simulink model "ENV_hardcoded"  (R2024b)
settings: Solver=FixedStepDiscrete  StartTime=0.0  StopTime=10.0  FixedStep=0.001  RelTol=1e-3
libraries: stm32blockslib x54, canmsglib x29, simulink x7, stm32f4xxblockslib x1
(part 3 of 5)

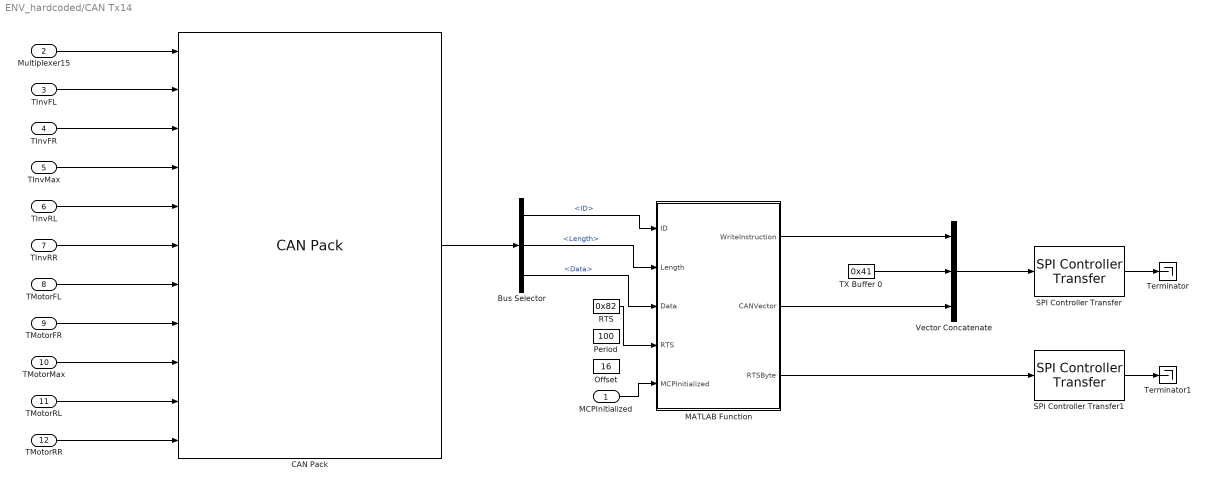
== system ENV_hardcoded/CAN Tx14 ==
  MCPInitialized : Inport  SampleTime=.001
  Multiplexer15 : Inport  Port=2
  TInvFL : Inport  Port=3
  TInvFR : Inport  Port=4
  TInvMax : Inport  Port=5
  TInvRL : Inport  Port=6
  TInvRR : Inport  Port=7
  TMotorFL : Inport  Port=8
  TMotorFR : Inport  Port=9
  TMotorMax : Inport  Port=10
  TMotorRL : Inport  Port=11
  TMotorRR : Inport  Port=12
  Bus Selector : BusSelector  OutputSignals=ID,Length,Data
  CAN Pack : canmsglib/CAN Pack  CANdbFile=C:\Users\William\Downloads\VCUSTM32\BaselineControls\CAN\CAN3_baseline.dbc  MsgList=Etas_Signals_15  MsgName=Etas_Signals_15  MsgIDType=Standard (11-bit identifier)  MsgIdentifier=2017  CANIDInput=off  MsgLength=8  Remote=off  ApplyMinMax=off  BusOutput=on  SignalInfo={'Multiplexer15','62','2','LE','unsigned','Multiplexor','0','1','0','0','3';'TInvFL','10','10','LE','unsigned','Multiplexed','1','0.1','0','0','102.3';'TInvFR','20','10','LE','unsigned','Multiplexed','1','0.1','0','0','102.3';'TInvMax','30','10','LE','unsigned','Multiplexed','1','0.1','0','0','102.3';'TInvRL','40','10','LE','unsigned','Multiplexed','1','0.1','0','0','102.3';'TInvRR','0','10','LE','unsigned','Multiplexed','1','0.1','0','0','102.3';'TMotorFL','12','11','LE','unsigned','Multiplexed','0','0.1','0','0','204.7';'TMotorFR','0','11','LE','unsigned','Multiplexed','0','0.1','0','0','204.7';'TMotorMax','45','11','LE','unsigned','Multiplexed','0','0.1','0','0','204.7';'TMotorRL','23','11','LE','unsigned','Multiplexed','0','0.1','0','0','204.7';'TMotorRR','34','11','LE','unsigned','Multiplexed','0','0.1','0','0','204.7'}
      settings: LibrarySourceBlock=stmutilitieslib/CAN Pack  DataFormat=CANdb specified signals
  MATLAB Function : MATLAB Function  TreatAsAtomicUnit=on
  Offset : Constant  Value=16  OutDataTypeStr=uint16  SampleTime=.001
  Period : Constant  Value=100  OutDataTypeStr=uint16  SampleTime=.001
  RTS : Constant  Value=0x82  OutDataTypeStr=uint8  SampleTime=.001
  SPI Controller Transfer : stm32blockslib/SPI Controller Transfer  Priority=1  SPIModuleSelect=SPI1  ClockPolarity=Low  ClockPhase=1 Edge  SPIModule=uint32(0)  Mode=Master  BusSpeed=uint32(1000000)  FirstBitToTransfer=Most significant bit (MSB)  ClockMode=0  BlockFunction=Transfer  EnableRegisterAddress=off  RegisterAddress=0  OutputDataType=uint8  OutputDataLength=1  OutputStatus=off  BlockingMode=off  Timeout=0.01  DataBits=8  UseCustomSSPin=Explicit GPIO calls  ActiveLowSSPin=Active low  Port_Select=GPIOA  Pin=4
      settings: LibrarySourceBlock=stm32h7xxblockslib/SPI Controller Transfer
  SPI Controller Transfer1 : stm32blockslib/SPI Controller Transfer  Priority=2  SPIModuleSelect=SPI1  ClockPolarity=Low  ClockPhase=1 Edge  SPIModule=uint32(0)  Mode=Master  BusSpeed=uint32(1000000)  FirstBitToTransfer=Most significant bit (MSB)  ClockMode=0  BlockFunction=Transfer  EnableRegisterAddress=off  RegisterAddress=0  OutputDataType=uint8  OutputDataLength=1  OutputStatus=off  BlockingMode=off  Timeout=0.01  DataBits=8  UseCustomSSPin=Explicit GPIO calls  ActiveLowSSPin=Active low  Port_Select=GPIOA  Pin=4
      settings: LibrarySourceBlock=stm32h7xxblockslib/SPI Controller Transfer
  TX Buffer 0 : Constant  Value=0x41  OutDataTypeStr=uint8  SampleTime=.001
  Terminator : Terminator
  Terminator1 : Terminator
  Vector Concatenate : Concatenate  NumInputs=3
  wires:
  TInvFL/1 -> CAN Pack/2
  Multiplexer15/1 -> CAN Pack/1
  TInvFR/1 -> CAN Pack/3
  TInvMax/1 -> CAN Pack/4
  TInvRL/1 -> CAN Pack/5
  TInvRR/1 -> CAN Pack/6
  TMotorFL/1 -> CAN Pack/7
  TMotorFR/1 -> CAN Pack/8
  TMotorMax/1 -> CAN Pack/9
  TMotorRL/1 -> CAN Pack/10
  TMotorRR/1 -> CAN Pack/11
  CAN Pack/1 -> Bus Selector/1
  SPI Controller Transfer/1 -> Terminator/1
  Bus Selector/1 -> MATLAB Function/1(ID)  "<ID>"
  Bus Selector/3 -> MATLAB Function/3(Data)  "<Data>"
  Vector Concatenate/1 -> SPI Controller Transfer/1
  Bus Selector/2 -> MATLAB Function/2(Length)  "<Length>"
  SPI Controller Transfer1/1 -> Terminator1/1
  MATLAB Function/2(CANVector) -> Vector Concatenate/3
  TX Buffer 0/1 -> Vector Concatenate/2
  MATLAB Function/3(RTSByte) -> SPI Controller Transfer1/1
  RTS/1 -> MATLAB Function/4(RTS)
  MCPInitialized/1 -> MATLAB Function/5(MCPInitialized)
  MATLAB Function/1(WriteInstruction) -> Vector Concatenate/1

== system ENV_hardcoded/CAN Tx15 ==
  MCPInitialized : Inport  SampleTime=.001
  NInvDTCFL : Inport  Port=2
  NInvDTCFR : Inport  Port=3
  NInvDTCRL : Inport  Port=4
  NInvDTCRR : Inport  Port=5
  TCellMax : Inport  Port=6
  VCellDelta : Inport  Port=7
  Bus Selector : BusSelector  OutputSignals=ID,Length,Data
  CAN Pack : canmsglib/CAN Pack  CANdbFile=C:\Users\William\Downloads\VCUSTM32\BaselineControls\CAN\CAN3_baseline.dbc  MsgList=Etas_Signals_16  MsgName=Etas_Signals_16  MsgIDType=Standard (11-bit identifier)  MsgIdentifier=2018  CANIDInput=off  MsgLength=8  Remote=off  ApplyMinMax=off  BusOutput=on  SignalInfo={'NInvDTCFL','12','12','LE','unsigned','Standard','0','1','0','0','4095';'NInvDTCFR','24','12','LE','unsigned','Standard','0','1','0','0','4095';'NinvDTCRL','36','12','LE','unsigned','Standard','0','1','0','0','4095';'NinvDTCRR','0','12','LE','unsigned','Standard','0','1','0','0','4095';'TCellMax','48','10','LE','unsigned','Standard','0','0.1','0','0','102.3';'VCellDelta','58','6','LE','unsigned','Standard','0','0.01','0','0','0.63'}
      settings: LibrarySourceBlock=stmutilitieslib/CAN Pack  DataFormat=CANdb specified signals
  MATLAB Function : MATLAB Function  TreatAsAtomicUnit=on
  Offset : Constant  Value=3  OutDataTypeStr=uint16  SampleTime=.001
  Period : Constant  Value=5  OutDataTypeStr=uint16  SampleTime=.001
  RTS : Constant  Value=0x81  OutDataTypeStr=uint8  SampleTime=.001
  SPI Controller Transfer : stm32blockslib/SPI Controller Transfer  Priority=1  SPIModuleSelect=SPI1  ClockPolarity=Low  ClockPhase=1 Edge  SPIModule=uint32(0)  Mode=Master  BusSpeed=uint32(1000000)  FirstBitToTransfer=Most significant bit (MSB)  ClockMode=0  BlockFunction=Transfer  EnableRegisterAddress=off  RegisterAddress=0  OutputDataType=uint8  OutputDataLength=1  OutputStatus=off  BlockingMode=off  Timeout=0.01  DataBits=8  UseCustomSSPin=Explicit GPIO calls  ActiveLowSSPin=Active low  Port_Select=GPIOA  Pin=4
      settings: LibrarySourceBlock=stm32h7xxblockslib/SPI Controller Transfer
  SPI Controller Transfer1 : stm32blockslib/SPI Controller Transfer  Priority=2  SPIModuleSelect=SPI1  ClockPolarity=Low  ClockPhase=1 Edge  SPIModule=uint32(0)  Mode=Master  BusSpeed=uint32(1000000)  FirstBitToTransfer=Most significant bit (MSB)  ClockMode=0  BlockFunction=Transfer  EnableRegisterAddress=off  RegisterAddress=0  OutputDataType=uint8  OutputDataLength=1  OutputStatus=off  BlockingMode=off  Timeout=0.01  DataBits=8  UseCustomSSPin=Explicit GPIO calls  ActiveLowSSPin=Active low  Port_Select=GPIOA  Pin=4
      settings: LibrarySourceBlock=stm32h7xxblockslib/SPI Controller Transfer
  TX Buffer 0 : Constant  Value=0x31  OutDataTypeStr=uint8  SampleTime=.001
  Terminator : Terminator
  Terminator1 : Terminator
  Vector Concatenate : Concatenate  NumInputs=3
  wires:
  NInvDTCFR/1 -> CAN Pack/2
  NInvDTCFL/1 -> CAN Pack/1
  NInvDTCRL/1 -> CAN Pack/3
  NInvDTCRR/1 -> CAN Pack/4
  TCellMax/1 -> CAN Pack/5
  VCellDelta/1 -> CAN Pack/6
  Bus Selector/2 -> MATLAB Function/2(Length)  "<Length>"
  MCPInitialized/1 -> MATLAB Function/5(MCPInitialized)
  Vector Concatenate/1 -> SPI Controller Transfer/1
  Bus Selector/3 -> MATLAB Function/3(Data)  "<Data>"
  MATLAB Function/3(RTSByte) -> SPI Controller Transfer1/1
  MATLAB Function/2(CANVector) -> Vector Concatenate/3
  Bus Selector/1 -> MATLAB Function/1(ID)  "<ID>"
  SPI Controller Transfer1/1 -> Terminator1/1
  SPI Controller Transfer/1 -> Terminator/1
  TX Buffer 0/1 -> Vector Concatenate/2
  MATLAB Function/1(WriteInstruction) -> Vector Concatenate/1
  RTS/1 -> MATLAB Function/4(RTS)
  CAN Pack/1 -> Bus Selector/1

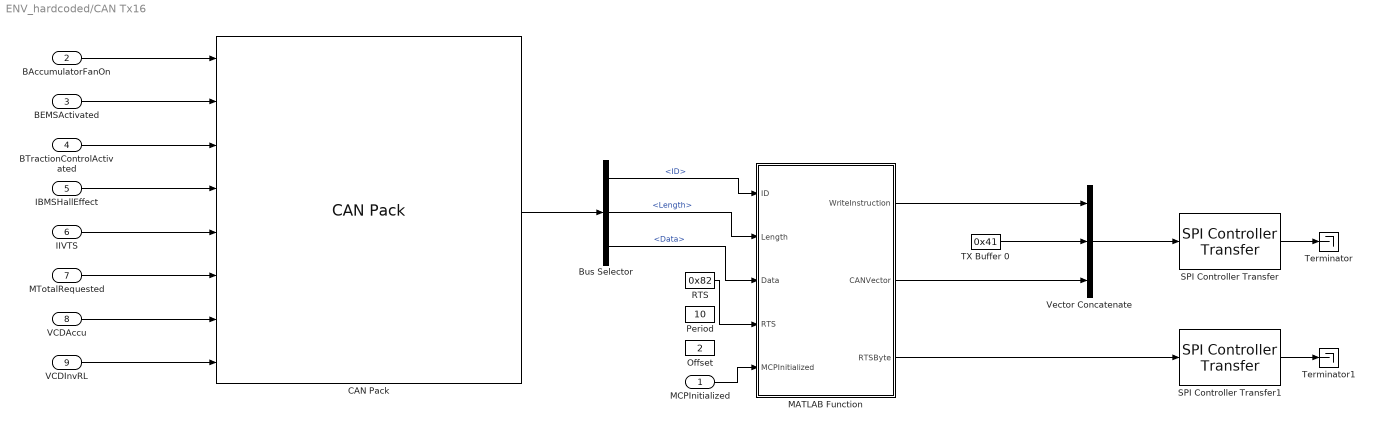
== system ENV_hardcoded/CAN Tx16 ==
  MCPInitialized : Inport  SampleTime=.001
  BAccumulatorFanOn : Inport  Port=2
  BEMSActivated : Inport  Port=3
  BTractionControlActivated : Inport  Port=4
  IBMSHallEffect : Inport  Port=5
  IIVTS : Inport  Port=6
  MTotalRequested : Inport  Port=7
  VCDAccu : Inport  Port=8
  VCDInvRL : Inport  Port=9
  Bus Selector : BusSelector  OutputSignals=ID,Length,Data
  CAN Pack : canmsglib/CAN Pack  CANdbFile=C:\Users\William\Downloads\VCUSTM32\BaselineControls\CAN\CAN3_baseline.dbc  MsgList=Etas_Signals_17  MsgName=Etas_Signals_17  MsgIDType=Standard (11-bit identifier)  MsgIdentifier=2019  CANIDInput=off  MsgLength=8  Remote=off  ApplyMinMax=off  BusOutput=on  SignalInfo={'BAccumulatorFanOn','63','1','LE','unsigned','Standard','0','1','0','0','1';'BEMSActivated','61','1','LE','unsigned','Standard','0','1','0','0','1';'BTractionControlActivated','62','1','LE','unsigned','Standard','0','1','0','0','1';'IBMSHallEffect','13','12','LE','signed','Standard','0','0.1','20','-184.8','224.7';'IIVTS','35','12','LE','signed','Standard','0','0.1','20','-184.8','224.7';'MTotalRequested','47','14','LE','signed','Standard','0','0.1','300','-519.2','1119.1';'VDCAccu','0','13','LE','unsigned','Standard','0','0.1','0','0','819.1';'VDCInvRL','25','10','LE','unsigned','Standard','0','1','0','0','1023'}
      settings: LibrarySourceBlock=stmutilitieslib/CAN Pack  DataFormat=CANdb specified signals
  MATLAB Function : MATLAB Function  TreatAsAtomicUnit=on
  Offset : Constant  Value=2  OutDataTypeStr=uint16  SampleTime=.001
  Period : Constant  Value=10  OutDataTypeStr=uint16  SampleTime=.001
  RTS : Constant  Value=0x82  OutDataTypeStr=uint8  SampleTime=.001
  SPI Controller Transfer : stm32blockslib/SPI Controller Transfer  Priority=1  SPIModuleSelect=SPI1  ClockPolarity=Low  ClockPhase=1 Edge  SPIModule=uint32(0)  Mode=Master  BusSpeed=uint32(1000000)  FirstBitToTransfer=Most significant bit (MSB)  ClockMode=0  BlockFunction=Transfer  EnableRegisterAddress=off  RegisterAddress=0  OutputDataType=uint8  OutputDataLength=1  OutputStatus=off  BlockingMode=off  Timeout=0.01  DataBits=8  UseCustomSSPin=Explicit GPIO calls  ActiveLowSSPin=Active low  Port_Select=GPIOA  Pin=4
      settings: LibrarySourceBlock=stm32h7xxblockslib/SPI Controller Transfer
  SPI Controller Transfer1 : stm32blockslib/SPI Controller Transfer  Priority=2  SPIModuleSelect=SPI1  ClockPolarity=Low  ClockPhase=1 Edge  SPIModule=uint32(0)  Mode=Master  BusSpeed=uint32(1000000)  FirstBitToTransfer=Most significant bit (MSB)  ClockMode=0  BlockFunction=Transfer  EnableRegisterAddress=off  RegisterAddress=0  OutputDataType=uint8  OutputDataLength=1  OutputStatus=off  BlockingMode=off  Timeout=0.01  DataBits=8  UseCustomSSPin=Explicit GPIO calls  ActiveLowSSPin=Active low  Port_Select=GPIOA  Pin=4
      settings: LibrarySourceBlock=stm32h7xxblockslib/SPI Controller Transfer
  TX Buffer 0 : Constant  Value=0x41  OutDataTypeStr=uint8  SampleTime=.001
  Terminator : Terminator
  Terminator1 : Terminator
  Vector Concatenate : Concatenate  NumInputs=3
  wires:
  BEMSActivated/1 -> CAN Pack/2
  BAccumulatorFanOn/1 -> CAN Pack/1
  BTractionControlActivated/1 -> CAN Pack/3
  IBMSHallEffect/1 -> CAN Pack/4
  IIVTS/1 -> CAN Pack/5
  MTotalRequested/1 -> CAN Pack/6
  VCDAccu/1 -> CAN Pack/7
  VCDInvRL/1 -> CAN Pack/8
  Bus Selector/2 -> MATLAB Function/2(Length)  "<Length>"
  Vector Concatenate/1 -> SPI Controller Transfer/1
  Bus Selector/1 -> MATLAB Function/1(ID)  "<ID>"
  SPI Controller Transfer/1 -> Terminator/1
  MATLAB Function/1(WriteInstruction) -> Vector Concatenate/1
  MATLAB Function/3(RTSByte) -> SPI Controller Transfer1/1
  RTS/1 -> MATLAB Function/4(RTS)
  SPI Controller Transfer1/1 -> Terminator1/1
  Bus Selector/3 -> MATLAB Function/3(Data)  "<Data>"
  MATLAB Function/2(CANVector) -> Vector Concatenate/3
  CAN Pack/1 -> Bus Selector/1
  TX Buffer 0/1 -> Vector Concatenate/2
  MCPInitialized/1 -> MATLAB Function/5(MCPInitialized)

== system ENV_hardcoded/CAN Tx17 ==
  MCPInitialized : Inport  SampleTime=.001
  NTractionControlKpSelector : Inport  Port=2
  TCellMin : Inport  Port=3
  TEtas : Inport  Port=4
  VCellMax : Inport  Port=5
  VCellMin : Inport  Port=6
  VLVSystem : Inport  Port=7
  tEtasOn : Inport  Port=8
  Bus Selector : BusSelector  OutputSignals=ID,Length,Data
  CAN Pack : canmsglib/CAN Pack  CANdbFile=C:\Users\William\Downloads\VCUSTM32\BaselineControls\CAN\CAN3_baseline.dbc  MsgList=Etas_Signals_18  MsgName=Etas_Signals_18  MsgIDType=Standard (11-bit identifier)  MsgIdentifier=2020  CANIDInput=off  MsgLength=8  Remote=off  ApplyMinMax=off  BusOutput=on  SignalInfo={'NTractionControlKpSelector','61','3','LE','unsigned','Standard','0','1','0','0','7';'TCellMin','18','10','LE','unsigned','Standard','0','0.1','0','0','102.3';'TEtas','36','10','LE','unsigned','Standard','0','0.1','0','0','102.3';'VCellMax','9','9','LE','unsigned','Standard','0','0.01','0','0','5.11';'VCellMin','0','9','LE','unsigned','Standard','0','0.01','0','0','5.11';'VLVSystem','28','8','LE','unsigned','Standard','0','0.1','0','0','25.5';'tEtasOn','46','15','LE','unsigned','Standard','0','0.1','0','0','3276.7'}
      settings: LibrarySourceBlock=stmutilitieslib/CAN Pack  DataFormat=CANdb specified signals
  MATLAB Function : MATLAB Function  TreatAsAtomicUnit=on
  Offset : Constant  Value=4  OutDataTypeStr=uint16  SampleTime=.001
  Period : Constant  Value=20  OutDataTypeStr=uint16  SampleTime=.001
  RTS : Constant  Value=0x82  OutDataTypeStr=uint8  SampleTime=.001
  SPI Controller Transfer : stm32blockslib/SPI Controller Transfer  Priority=1  SPIModuleSelect=SPI1  ClockPolarity=Low  ClockPhase=1 Edge  SPIModule=uint32(0)  Mode=Master  BusSpeed=uint32(1000000)  FirstBitToTransfer=Most significant bit (MSB)  ClockMode=0  BlockFunction=Transfer  EnableRegisterAddress=off  RegisterAddress=0  OutputDataType=uint8  OutputDataLength=1  OutputStatus=off  BlockingMode=off  Timeout=0.01  DataBits=8  UseCustomSSPin=Explicit GPIO calls  ActiveLowSSPin=Active low  Port_Select=GPIOA  Pin=4
      settings: LibrarySourceBlock=stm32h7xxblockslib/SPI Controller Transfer
  SPI Controller Transfer1 : stm32blockslib/SPI Controller Transfer  Priority=2  SPIModuleSelect=SPI1  ClockPolarity=Low  ClockPhase=1 Edge  SPIModule=uint32(0)  Mode=Master  BusSpeed=uint32(1000000)  FirstBitToTransfer=Most significant bit (MSB)  ClockMode=0  BlockFunction=Transfer  EnableRegisterAddress=off  RegisterAddress=0  OutputDataType=uint8  OutputDataLength=1  OutputStatus=off  BlockingMode=off  Timeout=0.01  DataBits=8  UseCustomSSPin=Explicit GPIO calls  ActiveLowSSPin=Active low  Port_Select=GPIOA  Pin=4
      settings: LibrarySourceBlock=stm32h7xxblockslib/SPI Controller Transfer
  TX Buffer 0 : Constant  Value=0x41  OutDataTypeStr=uint8  SampleTime=.001
  Terminator : Terminator
  Terminator1 : Terminator
  Vector Concatenate : Concatenate  NumInputs=3
  wires:
  TCellMin/1 -> CAN Pack/2
  NTractionControlKpSelector/1 -> CAN Pack/1
  TEtas/1 -> CAN Pack/3
  VCellMax/1 -> CAN Pack/4
  VCellMin/1 -> CAN Pack/5
  VLVSystem/1 -> CAN Pack/6
  tEtasOn/1 -> CAN Pack/7
  RTS/1 -> MATLAB Function/4(RTS)
  MATLAB Function/1(WriteInstruction) -> Vector Concatenate/1
  TX Buffer 0/1 -> Vector Concatenate/2
  SPI Controller Transfer1/1 -> Terminator1/1
  MATLAB Function/2(CANVector) -> Vector Concatenate/3
  Bus Selector/2 -> MATLAB Function/2(Length)  "<Length>"
  Bus Selector/3 -> MATLAB Function/3(Data)  "<Data>"
  Vector Concatenate/1 -> SPI Controller Transfer/1
  MCPInitialized/1 -> MATLAB Function/5(MCPInitialized)
  Bus Selector/1 -> MATLAB Function/1(ID)  "<ID>"
  CAN Pack/1 -> Bus Selector/1
  SPI Controller Transfer/1 -> Terminator/1
  MATLAB Function/3(RTSByte) -> SPI Controller Transfer1/1

== system ENV_hardcoded/CAN Tx18 ==
  MCPInitialized : Inport  SampleTime=.001
  PDischargeLimited : Inport  Port=2
  aSteeringAngle : Inport  Port=3
  nYawRateErrorActual : Inport  Port=4
  rRegenPaddle : Inport  Port=5
  rSplitRear : Inport  Port=6
  tAppsTimer : Inport  Port=7
  tPedalOverlap : Inport  Port=8
  Bus Selector : BusSelector  OutputSignals=ID,Length,Data
  CAN Pack : canmsglib/CAN Pack  CANdbFile=C:\Users\William\Downloads\VCUSTM32\BaselineControls\CAN\CAN3_baseline.dbc  MsgList=Etas_Signals_19  MsgName=Etas_Signals_19  MsgIDType=Standard (11-bit identifier)  MsgIdentifier=2021  CANIDInput=off  MsgLength=8  Remote=off  ApplyMinMax=off  BusOutput=on  SignalInfo={'PDischargeLimited','47','10','LE','unsigned','Standard','0','0.1','0','0','102.3';'aSteeringAngle','27','10','LE','signed','Standard','0','0.1','0','-51.2','51.1';'nYawRateErrorActual','0','14','LE','signed','Standard','0','0.01','0','-81.92','81.91';'rRegenPaddle','37','10','LE','unsigned','Standard','0','0.1','0','0','102.3';'rSplitRear','57','7','LE','unsigned','Standard','0','0.01','0','0','1.27';'tAppsTimer','20','7','LE','unsigned','Standard','0','0.01','0','0','1.27';'tPedalOverlap','14','6','LE','unsigned','Standard','0','0.1','0','0','6.3'}
      settings: LibrarySourceBlock=stmutilitieslib/CAN Pack  DataFormat=CANdb specified signals
  MATLAB Function : MATLAB Function  TreatAsAtomicUnit=on
  Offset : Constant  Value=3  OutDataTypeStr=uint16  SampleTime=.001
  Period : Constant  Value=10  OutDataTypeStr=uint16  SampleTime=.001
  RTS : Constant  Value=0x82  OutDataTypeStr=uint8  SampleTime=.001
  SPI Controller Transfer : stm32blockslib/SPI Controller Transfer  Priority=1  SPIModuleSelect=SPI1  ClockPolarity=Low  ClockPhase=1 Edge  SPIModule=uint32(0)  Mode=Master  BusSpeed=uint32(1000000)  FirstBitToTransfer=Most significant bit (MSB)  ClockMode=0  BlockFunction=Transfer  EnableRegisterAddress=off  RegisterAddress=0  OutputDataType=uint8  OutputDataLength=1  OutputStatus=off  BlockingMode=off  Timeout=0.01  DataBits=8  UseCustomSSPin=Explicit GPIO calls  ActiveLowSSPin=Active low  Port_Select=GPIOA  Pin=4
      settings: LibrarySourceBlock=stm32h7xxblockslib/SPI Controller Transfer
  SPI Controller Transfer1 : stm32blockslib/SPI Controller Transfer  Priority=2  SPIModuleSelect=SPI1  ClockPolarity=Low  ClockPhase=1 Edge  SPIModule=uint32(0)  Mode=Master  BusSpeed=uint32(1000000)  FirstBitToTransfer=Most significant bit (MSB)  ClockMode=0  BlockFunction=Transfer  EnableRegisterAddress=off  RegisterAddress=0  OutputDataType=uint8  OutputDataLength=1  OutputStatus=off  BlockingMode=off  Timeout=0.01  DataBits=8  UseCustomSSPin=Explicit GPIO calls  ActiveLowSSPin=Active low  Port_Select=GPIOA  Pin=4
      settings: LibrarySourceBlock=stm32h7xxblockslib/SPI Controller Transfer
  TX Buffer 0 : Constant  Value=0x41  OutDataTypeStr=uint8  SampleTime=.001
  Terminator : Terminator
  Terminator1 : Terminator
  Vector Concatenate : Concatenate  NumInputs=3
  wires:
  aSteeringAngle/1 -> CAN Pack/2
  PDischargeLimited/1 -> CAN Pack/1
  nYawRateErrorActual/1 -> CAN Pack/3
  rRegenPaddle/1 -> CAN Pack/4
  rSplitRear/1 -> CAN Pack/5
  tAppsTimer/1 -> CAN Pack/6
  tPedalOverlap/1 -> CAN Pack/7
  Bus Selector/2 -> MATLAB Function/2(Length)  "<Length>"
  Vector Concatenate/1 -> SPI Controller Transfer/1
  Bus Selector/1 -> MATLAB Function/1(ID)  "<ID>"
  SPI Controller Transfer/1 -> Terminator/1
  MATLAB Function/1(WriteInstruction) -> Vector Concatenate/1
  MATLAB Function/3(RTSByte) -> SPI Controller Transfer1/1
  RTS/1 -> MATLAB Function/4(RTS)
  SPI Controller Transfer1/1 -> Terminator1/1
  Bus Selector/3 -> MATLAB Function/3(Data)  "<Data>"
  MATLAB Function/2(CANVector) -> Vector Concatenate/3
  CAN Pack/1 -> Bus Selector/1
  TX Buffer 0/1 -> Vector Concatenate/2
  MCPInitialized/1 -> MATLAB Function/5(MCPInitialized)

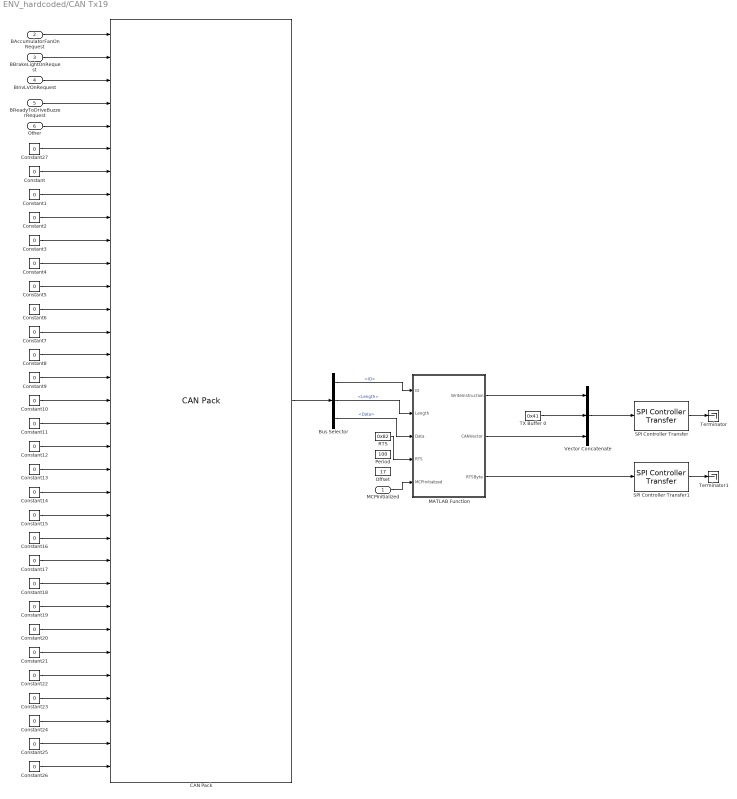
== system ENV_hardcoded/CAN Tx19 ==
  MCPInitialized : Inport  SampleTime=.001
  BAccumulatorFanOnRequest : Inport  Port=2
  BBrakeLightOnRequest : Inport  Port=3
  BInvLVOnRequest : Inport  Port=4
  BReadyToDriveBuzzerRequest : Inport  Port=5
  Other : Inport  Port=6
  Bus Selector : BusSelector  OutputSignals=ID,Length,Data
  CAN Pack : canmsglib/CAN Pack  CANdbFile=C:\Users\William\Downloads\VCUSTM32\BaselineControls\CAN\CAN3_baseline.dbc  MsgList=PDM_Req  MsgName=PDM_Req  MsgIDType=Standard (11-bit identifier)  MsgIdentifier=1536  CANIDInput=off  MsgLength=8  Remote=off  ApplyMinMax=off  BusOutput=on  SignalInfo={'BAccumulatorFanOnRequest','15','1','LE','unsigned','Standard','0','1','0','0','255';'BBrakeLightOnRequest','27','1','LE','unsigned','Standard','0','1','0','0','1';'BInvLVOnRequest','9','1','LE','unsigned','Standard','0','1','0','0','1';'BReadyToDriveBuzzerRequest','32','1','LE','unsigned','Standard','0','1','0','0','1';'C1P01','37','1','LE','unsigned','Standard','0','1','0','0','1';'C1P02','0','1','LE','unsigned','Standard','0','1','0','0','1';'C1P03','1','1','LE','unsigned','Standard','0','1','0','-Inf','Inf';'C1P04','2','1','LE','unsigned','Standard','0','1','0','0','1';'C1P07','38','1','LE','unsigned','Standard','0','1','0','0','1';'C1P11_Hbridge','39','2','LE','unsigned','Standard','0','1','0','0','3';'C1P13','3','1','LE','unsigned','Standard','0','1','0','0','1';'C1P25','5','1','LE','unsigned','Standard','0','1','0','0','1';'C1P28','7','1','LE','unsigned','Standard','0','1','0','0','1';'C1P30','8','1','LE','unsigned','Standard','0','1','0','0','1';'C1P33','10','1','LE','unsigned','Standard','0','1','0','0','1';'C1P34','11','1','LE','unsigned','Standard','0','1','0','0','1';'C1P36','41','1','LE','unsigned','Standard','0','1','0','0','1';'C1P37','42','1','LE','unsigned','Standard','0','1','0','0','1';'C1P38','13','1','LE','unsigned','Standard','0','1','0','-Inf','Inf';'C2P01','14','1','LE','unsigned','Standard','0','1','0','-Inf','Inf';'C2P03','24','1','LE','unsigned','Standard','0','1','0','-Inf','Inf';'C2P04','16','1','LE','unsigned','Standard','0','1','0','0','1';'C2P05','17','1','LE','unsigned','Standard','0','1','0','-Inf','Inf';'C2P25','36','1','LE','unsigned','Standard','0','1','0','0','1';'C2P26','22','1','LE','unsigned','Standard','0','1','0','-Inf','Inf';'C2P27','23','1','LE','unsigned','Standard','0','1','0','-Inf','Inf';'C2P28','25','1','LE','unsigned','Standard','0','1','0','-Inf','Inf';'C2P29','26','1','LE','unsigned','Standard','0','1','0','0','1';'C2P31','28','1','LE','unsigned','Standard','0','1','0','0','1';'C2P33','30','1','LE','unsigned','Standard','0','1','0','0','1';'C2P36','33','1','LE','unsigned','Standard','0','1','0','0','1';'C2P37','34','1','LE','unsigned','Standard','0','1','0','-Inf','Inf';'C2P38','35','1','LE','unsigned','Standard','0','1','0','-Inf','Inf'}
      settings: LibrarySourceBlock=stmutilitieslib/CAN Pack  DataFormat=CANdb specified signals
  Constant{,1..27} (28 alike) : Constant  Value=0
  MATLAB Function : MATLAB Function  TreatAsAtomicUnit=on
  Offset : Constant  Value=17  OutDataTypeStr=uint16  SampleTime=.001
  Period : Constant  Value=100  OutDataTypeStr=uint16  SampleTime=.001
  RTS : Constant  Value=0x82  OutDataTypeStr=uint8  SampleTime=.001
  SPI Controller Transfer : stm32blockslib/SPI Controller Transfer  Priority=1  SPIModuleSelect=SPI1  ClockPolarity=Low  ClockPhase=1 Edge  SPIModule=uint32(0)  Mode=Master  BusSpeed=uint32(1000000)  FirstBitToTransfer=Most significant bit (MSB)  ClockMode=0  BlockFunction=Transfer  EnableRegisterAddress=off  RegisterAddress=0  OutputDataType=uint8  OutputDataLength=1  OutputStatus=off  BlockingMode=off  Timeout=0.01  DataBits=8  UseCustomSSPin=Explicit GPIO calls  ActiveLowSSPin=Active low  Port_Select=GPIOA  Pin=4
      settings: LibrarySourceBlock=stm32h7xxblockslib/SPI Controller Transfer
  SPI Controller Transfer1 : stm32blockslib/SPI Controller Transfer  Priority=2  SPIModuleSelect=SPI1  ClockPolarity=Low  ClockPhase=1 Edge  SPIModule=uint32(0)  Mode=Master  BusSpeed=uint32(1000000)  FirstBitToTransfer=Most significant bit (MSB)  ClockMode=0  BlockFunction=Transfer  EnableRegisterAddress=off  RegisterAddress=0  OutputDataType=uint8  OutputDataLength=1  OutputStatus=off  BlockingMode=off  Timeout=0.01  DataBits=8  UseCustomSSPin=Explicit GPIO calls  ActiveLowSSPin=Active low  Port_Select=GPIOA  Pin=4
      settings: LibrarySourceBlock=stm32h7xxblockslib/SPI Controller Transfer
  TX Buffer 0 : Constant  Value=0x41  OutDataTypeStr=uint8  SampleTime=.001
  Terminator : Terminator
  Terminator1 : Terminator
  Vector Concatenate : Concatenate  NumInputs=3
  wires:
  BBrakeLightOnRequest/1 -> CAN Pack/2
  BAccumulatorFanOnRequest/1 -> CAN Pack/1
  BInvLVOnRequest/1 -> CAN Pack/3
  BReadyToDriveBuzzerRequest/1 -> CAN Pack/4
  Other/1 -> CAN Pack/5
  Constant27/1 -> CAN Pack/6
  Constant/1 -> CAN Pack/7
  Constant1/1 -> CAN Pack/8
  Constant7/1 -> CAN Pack/14
  Constant26/1 -> CAN Pack/33
  Constant25/1 -> CAN Pack/32
  Constant24/1 -> CAN Pack/31
  Constant23/1 -> CAN Pack/30
  Constant22/1 -> CAN Pack/29
  Constant21/1 -> CAN Pack/28
  Constant20/1 -> CAN Pack/27
  Constant19/1 -> CAN Pack/26
  Constant18/1 -> CAN Pack/25
  Constant17/1 -> CAN Pack/24
  Constant16/1 -> CAN Pack/23
  Constant15/1 -> CAN Pack/22
  Constant14/1 -> CAN Pack/21
  Constant13/1 -> CAN Pack/20
  Constant12/1 -> CAN Pack/19
  Constant11/1 -> CAN Pack/18
  Constant10/1 -> CAN Pack/17
  Constant9/1 -> CAN Pack/16
  Constant8/1 -> CAN Pack/15
  Constant6/1 -> CAN Pack/13
  Constant5/1 -> CAN Pack/12
  Constant4/1 -> CAN Pack/11
  Constant3/1 -> CAN Pack/10
  Constant2/1 -> CAN Pack/9
  Bus Selector/2 -> MATLAB Function/2(Length)  "<Length>"
  Vector Concatenate/1 -> SPI Controller Transfer/1
  Bus Selector/1 -> MATLAB Function/1(ID)  "<ID>"
  SPI Controller Transfer/1 -> Terminator/1
  MATLAB Function/1(WriteInstruction) -> Vector Concatenate/1
  MATLAB Function/3(RTSByte) -> SPI Controller Transfer1/1
  RTS/1 -> MATLAB Function/4(RTS)
  SPI Controller Transfer1/1 -> Terminator1/1
  Bus Selector/3 -> MATLAB Function/3(Data)  "<Data>"
  MATLAB Function/2(CANVector) -> Vector Concatenate/3
  CAN Pack/1 -> Bus Selector/1
  TX Buffer 0/1 -> Vector Concatenate/2
  MCPInitialized/1 -> MATLAB Function/5(MCPInitialized)

== system ENV_hardcoded/CAN Tx2 ==
  MCPInitialized : Inport  SampleTime=.001
  rSOETargetError : Inport  Port=2
  sEMS1000m : Inport  Port=3
  vWheelFL : Inport  Port=4
  vWheelFR : Inport  Port=5
  vWheelRL : Inport  Port=6
  vWheelRR : Inport  Port=7
  Bus Selector : BusSelector  OutputSignals=ID,Length,Data
  CAN Pack : canmsglib/CAN Pack  CANdbFile=C:\Users\William\Downloads\VCUSTM32\BaselineControls\CAN\CAN3_baseline.dbc  MsgList=Etas_Signals_03  MsgName=Etas_Signals_03  MsgIDType=Standard (11-bit identifier)  MsgIdentifier=2024  CANIDInput=off  MsgLength=8  Remote=off  ApplyMinMax=off  BusOutput=on  SignalInfo={'rSOETargetError','10','13','LE','signed','Standard','0','0.001','0','-4.096','4.095';'sEMS1000m','0','10','LE','unsigned','Standard','0','1','0','0','1023';'vWheelFL','24','8','LE','unsigned','Standard','0','0.1','0','0','25.5';'vWheelFR','32','8','LE','unsigned','Standard','0','0.1','0','0','25.5';'vWheelRL','40','8','LE','unsigned','Standard','0','0.1','0','0','25.5';'vWheelRR','48','8','LE','unsigned','Standard','0','0.1','0','0','25.5'}
      settings: LibrarySourceBlock=stmutilitieslib/CAN Pack  DataFormat=CANdb specified signals
  MATLAB Function : MATLAB Function  TreatAsAtomicUnit=on
  Offset : Constant  Value=15  OutDataTypeStr=uint16  SampleTime=.001
  Period : Constant  Value=100  OutDataTypeStr=uint16  SampleTime=.001
  RTS : Constant  Value=0x82  OutDataTypeStr=uint8  SampleTime=.001
  SPI Controller Transfer : stm32blockslib/SPI Controller Transfer  Priority=1  SPIModuleSelect=SPI1  ClockPolarity=Low  ClockPhase=1 Edge  SPIModule=uint32(0)  Mode=Master  BusSpeed=uint32(1000000)  FirstBitToTransfer=Most significant bit (MSB)  ClockMode=0  BlockFunction=Transfer  EnableRegisterAddress=off  RegisterAddress=0  OutputDataType=uint8  OutputDataLength=1  OutputStatus=off  BlockingMode=off  Timeout=0.01  DataBits=8  UseCustomSSPin=Explicit GPIO calls  ActiveLowSSPin=Active low  Port_Select=GPIOA  Pin=4
      settings: LibrarySourceBlock=stm32h7xxblockslib/SPI Controller Transfer
  SPI Controller Transfer1 : stm32blockslib/SPI Controller Transfer  Priority=2  SPIModuleSelect=SPI1  ClockPolarity=Low  ClockPhase=1 Edge  SPIModule=uint32(0)  Mode=Master  BusSpeed=uint32(1000000)  FirstBitToTransfer=Most significant bit (MSB)  ClockMode=0  BlockFunction=Transfer  EnableRegisterAddress=off  RegisterAddress=0  OutputDataType=uint8  OutputDataLength=1  OutputStatus=off  BlockingMode=off  Timeout=0.01  DataBits=8  UseCustomSSPin=Explicit GPIO calls  ActiveLowSSPin=Active low  Port_Select=GPIOA  Pin=4
      settings: LibrarySourceBlock=stm32h7xxblockslib/SPI Controller Transfer
  TX Buffer 0 : Constant  Value=0x41  OutDataTypeStr=uint8  SampleTime=.001
  Terminator : Terminator
  Terminator1 : Terminator
  Vector Concatenate : Concatenate  NumInputs=3
  wires:
  sEMS1000m/1 -> CAN Pack/2
  rSOETargetError/1 -> CAN Pack/1
  vWheelFL/1 -> CAN Pack/3
  vWheelFR/1 -> CAN Pack/4
  vWheelRL/1 -> CAN Pack/5
  vWheelRR/1 -> CAN Pack/6
  CAN Pack/1 -> Bus Selector/1
  SPI Controller Transfer/1 -> Terminator/1
  Bus Selector/1 -> MATLAB Function/1(ID)  "<ID>"
  Bus Selector/3 -> MATLAB Function/3(Data)  "<Data>"
  Vector Concatenate/1 -> SPI Controller Transfer/1
  Bus Selector/2 -> MATLAB Function/2(Length)  "<Length>"
  SPI Controller Transfer1/1 -> Terminator1/1
  MATLAB Function/2(CANVector) -> Vector Concatenate/3
  TX Buffer 0/1 -> Vector Concatenate/2
  MATLAB Function/3(RTSByte) -> SPI Controller Transfer1/1
  RTS/1 -> MATLAB Function/4(RTS)
  MCPInitialized/1 -> MATLAB Function/5(MCPInitialized)
  MATLAB Function/1(WriteInstruction) -> Vector Concatenate/1

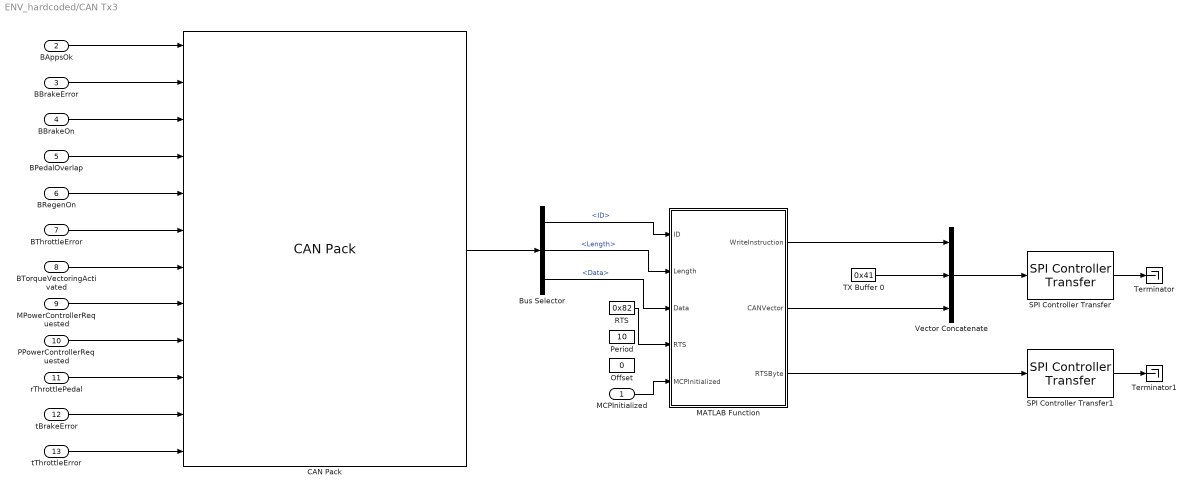
== system ENV_hardcoded/CAN Tx3 ==
  MCPInitialized : Inport  SampleTime=.001
  BAppsOk : Inport  Port=2
  BBrakeError : Inport  Port=3
  BBrakeOn : Inport  Port=4
  BPedalOverlap : Inport  Port=5
  BRegenOn : Inport  Port=6
  BThrottleError : Inport  Port=7
  BTorqueVectoringActivated : Inport  Port=8
  MPowerControllerRequested : Inport  Port=9
  PPowerControllerRequested : Inport  Port=10
  rThrottlePedal : Inport  Port=11
  tBrakeError : Inport  Port=12
  tThrottleError : Inport  Port=13
  Bus Selector : BusSelector  OutputSignals=ID,Length,Data
  CAN Pack : canmsglib/CAN Pack  CANdbFile=C:\Users\William\Downloads\VCUSTM32\BaselineControls\CAN\CAN3_baseline.dbc  MsgList=Etas_Signals_04  MsgName=Etas_Signals_04  MsgIDType=Standard (11-bit identifier)  MsgIdentifier=2025  CANIDInput=off  MsgLength=8  Remote=off  ApplyMinMax=off  BusOutput=on  SignalInfo={'BAppsOk','61','1','LE','unsigned','Standard','0','1','0','0','1';'BBrakeError','50','1','LE','unsigned','Standard','0','1','0','0','1';'BBrakeOn','59','1','LE','unsigned','Standard','0','1','0','0','1';'BPedalOverlap','60','1','LE','unsigned','Standard','0','1','0','0','1';'BRegenOn','62','1','LE','unsigned','Standard','0','1','0','0','1';'BThrottleError','41','1','LE','unsigned','Standard','0','1','0','0','1';'BTorqueVectoringActivated','63','1','LE','unsigned','Standard','0','1','0','0','1';'MPowerControllerRequested','14','17','LE','signed','Standard','0','0.01','300','-355.36','955.35';'PPowerControllerRequested','0','14','LE','signed','Standard','0','0.01','30','-51.92','111.91';'rThrottlePedal','31','10','LE','unsigned','Standard','0','0.1','0','0','102.3';'tBrakeError','51','8','LE','unsigned','Standard','0','0.1','0','0','25.5';'tThrottleError','42','8','LE','unsigned','Standard','0','0.1','0','0','25.5'}
      settings: LibrarySourceBlock=stmutilitieslib/CAN Pack  DataFormat=CANdb specified signals
  MATLAB Function : MATLAB Function  TreatAsAtomicUnit=on
  Offset : Constant  Value=0  OutDataTypeStr=uint16  SampleTime=.001
  Period : Constant  Value=10  OutDataTypeStr=uint16  SampleTime=.001
  RTS : Constant  Value=0x82  OutDataTypeStr=uint8  SampleTime=.001
  SPI Controller Transfer : stm32blockslib/SPI Controller Transfer  Priority=1  SPIModuleSelect=SPI1  ClockPolarity=Low  ClockPhase=1 Edge  SPIModule=uint32(0)  Mode=Master  BusSpeed=uint32(1000000)  FirstBitToTransfer=Most significant bit (MSB)  ClockMode=0  BlockFunction=Transfer  EnableRegisterAddress=off  RegisterAddress=0  OutputDataType=uint8  OutputDataLength=1  OutputStatus=off  BlockingMode=off  Timeout=0.01  DataBits=8  UseCustomSSPin=Explicit GPIO calls  ActiveLowSSPin=Active low  Port_Select=GPIOA  Pin=4
      settings: LibrarySourceBlock=stm32h7xxblockslib/SPI Controller Transfer
  SPI Controller Transfer1 : stm32blockslib/SPI Controller Transfer  Priority=2  SPIModuleSelect=SPI1  ClockPolarity=Low  ClockPhase=1 Edge  SPIModule=uint32(0)  Mode=Master  BusSpeed=uint32(1000000)  FirstBitToTransfer=Most significant bit (MSB)  ClockMode=0  BlockFunction=Transfer  EnableRegisterAddress=off  RegisterAddress=0  OutputDataType=uint8  OutputDataLength=1  OutputStatus=off  BlockingMode=off  Timeout=0.01  DataBits=8  UseCustomSSPin=Explicit GPIO calls  ActiveLowSSPin=Active low  Port_Select=GPIOA  Pin=4
      settings: LibrarySourceBlock=stm32h7xxblockslib/SPI Controller Transfer
  TX Buffer 0 : Constant  Value=0x41  OutDataTypeStr=uint8  SampleTime=.001
  Terminator : Terminator
  Terminator1 : Terminator
  Vector Concatenate : Concatenate  NumInputs=3
  wires:
  BBrakeError/1 -> CAN Pack/2
  BAppsOk/1 -> CAN Pack/1
  BBrakeOn/1 -> CAN Pack/3
  BPedalOverlap/1 -> CAN Pack/4
  BRegenOn/1 -> CAN Pack/5
  BThrottleError/1 -> CAN Pack/6
  BTorqueVectoringActivated/1 -> CAN Pack/7
  MPowerControllerRequested/1 -> CAN Pack/8
  PPowerControllerRequested/1 -> CAN Pack/9
  rThrottlePedal/1 -> CAN Pack/10
  tBrakeError/1 -> CAN Pack/11
  tThrottleError/1 -> CAN Pack/12
  CAN Pack/1 -> Bus Selector/1
  SPI Controller Transfer/1 -> Terminator/1
  Bus Selector/1 -> MATLAB Function/1(ID)  "<ID>"
  Bus Selector/3 -> MATLAB Function/3(Data)  "<Data>"
  Vector Concatenate/1 -> SPI Controller Transfer/1
  Bus Selector/2 -> MATLAB Function/2(Length)  "<Length>"
  SPI Controller Transfer1/1 -> Terminator1/1
  MATLAB Function/2(CANVector) -> Vector Concatenate/3
  TX Buffer 0/1 -> Vector Concatenate/2
  MATLAB Function/3(RTSByte) -> SPI Controller Transfer1/1
  RTS/1 -> MATLAB Function/4(RTS)
  MCPInitialized/1 -> MATLAB Function/5(MCPInitialized)
  MATLAB Function/1(WriteInstruction) -> Vector Concatenate/1

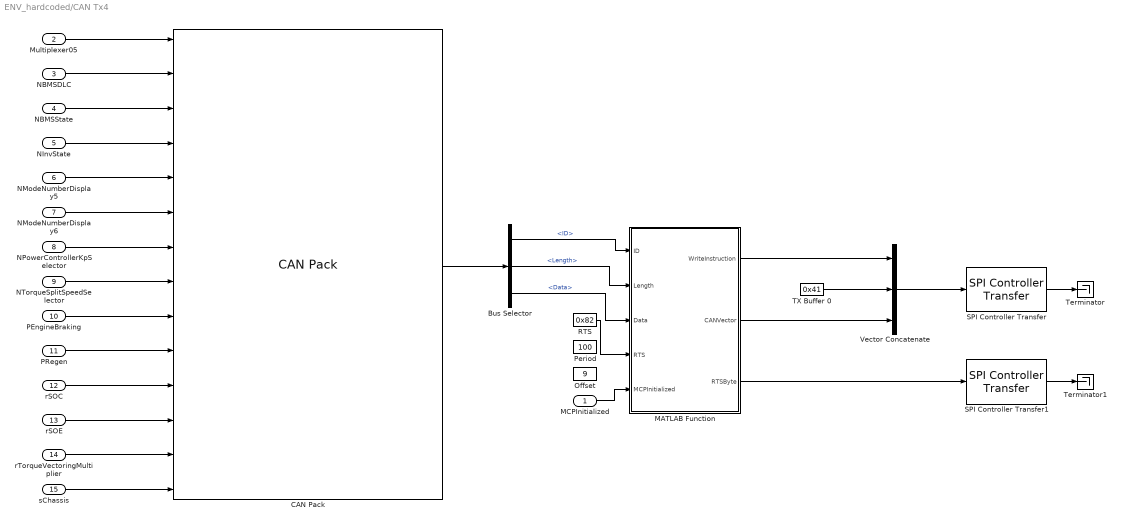
== system ENV_hardcoded/CAN Tx4 ==
  MCPInitialized : Inport  SampleTime=.001
  Multiplexer05 : Inport  Port=2
  NBMSDLC : Inport  Port=3
  NBMSState : Inport  Port=4
  NInvState : Inport  Port=5
  NModeNumberDisplay5 : Inport  Port=6
  NModeNumberDisplay6 : Inport  Port=7
  NPowerControllerKpSelector : Inport  Port=8
  NTorqueSplitSpeedSelector : Inport  Port=9
  PEngineBraking : Inport  Port=10
  PRegen : Inport  Port=11
  rSOC : Inport  Port=12
  rSOE : Inport  Port=13
  rTorqueVectoringMultiplier : Inport  Port=14
  sChassis : Inport  Port=15
  Bus Selector : BusSelector  OutputSignals=ID,Length,Data
  CAN Pack : canmsglib/CAN Pack  CANdbFile=C:\Users\William\Downloads\VCUSTM32\BaselineControls\CAN\CAN3_baseline.dbc  MsgList=Etas_Signals_05  MsgName=Etas_Signals_05  MsgIDType=Standard (11-bit identifier)  MsgIdentifier=2033  CANIDInput=off  MsgLength=8  Remote=off  ApplyMinMax=off  BusOutput=on  SignalInfo={'Multiplexer05','63','1','LE','unsigned','Multiplexor','0','1','0','0','511';'NBMSDLC','37','1','LE','unsigned','Multiplexed','0','1','0','0','1';'NBMSState','36','7','LE','unsigned','Multiplexed','1','1','0','0','127';'NInvState','43','9','LE','unsigned','Multiplexed','1','1','0','0','511';'NModeNumberDisplay5','28','4','LE','unsigned','Multiplexed','1','1','0','0','15';'NModeNumberDisplay6','32','4','LE','unsigned','Multiplexed','1','1','0','0','15';'NPowerControllerKpSelector','33','3','LE','unsigned','Multiplexed','0','1','0','0','7';'NTorqueSplitSpeedSelector','36','1','LE','unsigned','Multiplexed','0','1','1','1','2';'PEngineBraking','28','5','LE','unsigned','Multiplexed','0','1','0','0','31';'PRegen','15','6','LE','unsigned','Multiplexed','1','1','0','0','63';'rSOC','14','14','LE','unsigned','Multiplexed','0','0.01','0','0','163.83';'rSOE','0','14','LE','unsigned','Multiplexed','0','0.01','0','0','163.83';'rTorqueVectoringMultiplier','21','7','LE','unsigned','Multiplexed','1','0.01','0','0','1.27';'sChassis','0','15','LE','unsigned','Multiplexed','1','1','0','0','32767'}
      settings: LibrarySourceBlock=stmutilitieslib/CAN Pack  DataFormat=CANdb specified signals
  MATLAB Function : MATLAB Function  TreatAsAtomicUnit=on
  Offset : Constant  Value=9  OutDataTypeStr=uint16  SampleTime=.001
  Period : Constant  Value=100  OutDataTypeStr=uint16  SampleTime=.001
  RTS : Constant  Value=0x82  OutDataTypeStr=uint8  SampleTime=.001
  SPI Controller Transfer : stm32blockslib/SPI Controller Transfer  Priority=1  SPIModuleSelect=SPI1  ClockPolarity=Low  ClockPhase=1 Edge  SPIModule=uint32(0)  Mode=Master  BusSpeed=uint32(1000000)  FirstBitToTransfer=Most significant bit (MSB)  ClockMode=0  BlockFunction=Transfer  EnableRegisterAddress=off  RegisterAddress=0  OutputDataType=uint8  OutputDataLength=1  OutputStatus=off  BlockingMode=off  Timeout=0.01  DataBits=8  UseCustomSSPin=Explicit GPIO calls  ActiveLowSSPin=Active low  Port_Select=GPIOA  Pin=4
      settings: LibrarySourceBlock=stm32h7xxblockslib/SPI Controller Transfer
  SPI Controller Transfer1 : stm32blockslib/SPI Controller Transfer  Priority=2  SPIModuleSelect=SPI1  ClockPolarity=Low  ClockPhase=1 Edge  SPIModule=uint32(0)  Mode=Master  BusSpeed=uint32(1000000)  FirstBitToTransfer=Most significant bit (MSB)  ClockMode=0  BlockFunction=Transfer  EnableRegisterAddress=off  RegisterAddress=0  OutputDataType=uint8  OutputDataLength=1  OutputStatus=off  BlockingMode=off  Timeout=0.01  DataBits=8  UseCustomSSPin=Explicit GPIO calls  ActiveLowSSPin=Active low  Port_Select=GPIOA  Pin=4
      settings: LibrarySourceBlock=stm32h7xxblockslib/SPI Controller Transfer
  TX Buffer 0 : Constant  Value=0x41  OutDataTypeStr=uint8  SampleTime=.001
  Terminator : Terminator
  Terminator1 : Terminator
  Vector Concatenate : Concatenate  NumInputs=3
  wires:
  NBMSDLC/1 -> CAN Pack/2
  Multiplexer05/1 -> CAN Pack/1
  NBMSState/1 -> CAN Pack/3
  NInvState/1 -> CAN Pack/4
  NModeNumberDisplay5/1 -> CAN Pack/5
  NModeNumberDisplay6/1 -> CAN Pack/6
  NPowerControllerKpSelector/1 -> CAN Pack/7
  NTorqueSplitSpeedSelector/1 -> CAN Pack/8
  PEngineBraking/1 -> CAN Pack/9
  PRegen/1 -> CAN Pack/10
  rSOC/1 -> CAN Pack/11
  rSOE/1 -> CAN Pack/12
  sChassis/1 -> CAN Pack/14
  rTorqueVectoringMultiplier/1 -> CAN Pack/13
  Bus Selector/2 -> MATLAB Function/2(Length)  "<Length>"
  Vector Concatenate/1 -> SPI Controller Transfer/1
  Bus Selector/1 -> MATLAB Function/1(ID)  "<ID>"
  SPI Controller Transfer/1 -> Terminator/1
  MATLAB Function/1(WriteInstruction) -> Vector Concatenate/1
  MATLAB Function/3(RTSByte) -> SPI Controller Transfer1/1
  RTS/1 -> MATLAB Function/4(RTS)
  SPI Controller Transfer1/1 -> Terminator1/1
  Bus Selector/3 -> MATLAB Function/3(Data)  "<Data>"
  MATLAB Function/2(CANVector) -> Vector Concatenate/3
  CAN Pack/1 -> Bus Selector/1
  TX Buffer 0/1 -> Vector Concatenate/2
  MCPInitialized/1 -> MATLAB Function/5(MCPInitialized)

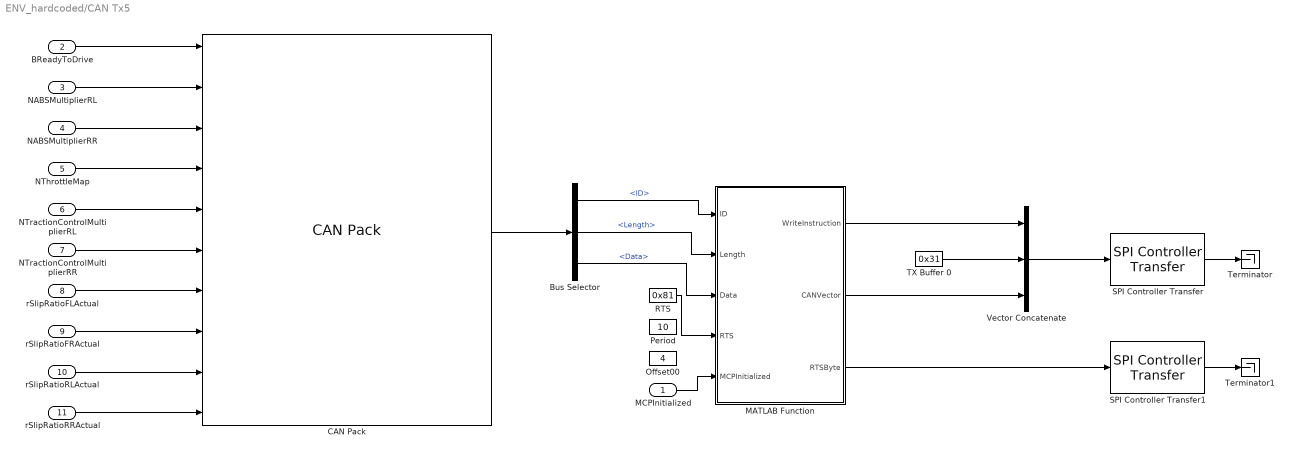
== system ENV_hardcoded/CAN Tx5 ==
  MCPInitialized : Inport  SampleTime=.001
  BReadyToDrive : Inport  Port=2
  NABSMultiplierRL : Inport  Port=3
  NABSMultiplierRR : Inport  Port=4
  NThrottleMap : Inport  Port=5
  NTractionControlMultiplierRL : Inport  Port=6
  NTractionControlMultiplierRR : Inport  Port=7
  rSlipRatioFLActual : Inport  Port=8
  rSlipRatioFRActual : Inport  Port=9
  rSlipRatioRLActual : Inport  Port=10
  rSlipRatioRRActual : Inport  Port=11
  Bus Selector : BusSelector  OutputSignals=ID,Length,Data
  CAN Pack : canmsglib/CAN Pack  CANdbFile=C:\Users\William\Downloads\VCUSTM32\BaselineControls\CAN\CAN3_baseline.dbc  MsgList=Etas_Signals_06  MsgName=Etas_Signals_06  MsgIDType=Standard (11-bit identifier)  MsgIdentifier=2034  CANIDInput=off  MsgLength=8  Remote=off  ApplyMinMax=off  BusOutput=on  SignalInfo={'BReadyToDrive','63','1','LE','unsigned','Standard','0','1','0','0','1';'NABSMultiplierRL','53','7','LE','unsigned','Standard','0','0.01','0','0','1.27';'NABSMultiplierRR','39','7','LE','unsigned','Standard','0','0.01','0','0','1.27';'NThrottleMap','60','3','LE','unsigned','Standard','0','1','0','0','7';'NTractionControlMultiplierRL','46','7','LE','unsigned','Standard','0','0.01','0','0','1.27';'NTractionControlMultiplierRR','32','7','LE','unsigned','Standard','0','0.01','0','0','1.27';'rSlipRatioFLActual','24','8','LE','signed','Standard','0','0.01','0','-1.28','1.27';'rSlipRatioFRActual','16','8','LE','signed','Standard','0','0.01','0','-1.28','1.27';'rSlipRatioRLActual','8','8','LE','signed','Standard','0','0.01','0','-1.28','1.27';'rSlipRatioRRActual','0','8','LE','signed','Standard','0','0.01','0','-1.28','1.27'}
      settings: LibrarySourceBlock=stmutilitieslib/CAN Pack  DataFormat=CANdb specified signals
  MATLAB Function : MATLAB Function  TreatAsAtomicUnit=on
  Offset00 : Constant  Value=4  OutDataTypeStr=uint16  SampleTime=.001
  Period : Constant  Value=10  OutDataTypeStr=uint16  SampleTime=.001
  RTS : Constant  Value=0x81  OutDataTypeStr=uint8  SampleTime=.001
  SPI Controller Transfer : stm32blockslib/SPI Controller Transfer  Priority=1  SPIModuleSelect=SPI1  ClockPolarity=Low  ClockPhase=1 Edge  SPIModule=uint32(0)  Mode=Master  BusSpeed=uint32(1000000)  FirstBitToTransfer=Most significant bit (MSB)  ClockMode=0  BlockFunction=Transfer  EnableRegisterAddress=off  RegisterAddress=0  OutputDataType=uint8  OutputDataLength=1  OutputStatus=off  BlockingMode=off  Timeout=0.01  DataBits=8  UseCustomSSPin=Explicit GPIO calls  ActiveLowSSPin=Active low  Port_Select=GPIOA  Pin=4
      settings: LibrarySourceBlock=stm32h7xxblockslib/SPI Controller Transfer
  SPI Controller Transfer1 : stm32blockslib/SPI Controller Transfer  Priority=2  SPIModuleSelect=SPI1  ClockPolarity=Low  ClockPhase=1 Edge  SPIModule=uint32(0)  Mode=Master  BusSpeed=uint32(1000000)  FirstBitToTransfer=Most significant bit (MSB)  ClockMode=0  BlockFunction=Transfer  EnableRegisterAddress=off  RegisterAddress=0  OutputDataType=uint8  OutputDataLength=1  OutputStatus=off  BlockingMode=off  Timeout=0.01  DataBits=8  UseCustomSSPin=Explicit GPIO calls  ActiveLowSSPin=Active low  Port_Select=GPIOA  Pin=4
      settings: LibrarySourceBlock=stm32h7xxblockslib/SPI Controller Transfer
  TX Buffer 0 : Constant  Value=0x31  OutDataTypeStr=uint8  SampleTime=.001
  Terminator : Terminator
  Terminator1 : Terminator
  Vector Concatenate : Concatenate  NumInputs=3
  wires:
  NABSMultiplierRL/1 -> CAN Pack/2
  BReadyToDrive/1 -> CAN Pack/1
  NABSMultiplierRR/1 -> CAN Pack/3
  NThrottleMap/1 -> CAN Pack/4
  NTractionControlMultiplierRL/1 -> CAN Pack/5
  NTractionControlMultiplierRR/1 -> CAN Pack/6
  rSlipRatioFLActual/1 -> CAN Pack/7
  rSlipRatioFRActual/1 -> CAN Pack/8
  rSlipRatioRLActual/1 -> CAN Pack/9
  rSlipRatioRRActual/1 -> CAN Pack/10
  CAN Pack/1 -> Bus Selector/1
  SPI Controller Transfer/1 -> Terminator/1
  Bus Selector/1 -> MATLAB Function/1(ID)  "<ID>"
  Bus Selector/3 -> MATLAB Function/3(Data)  "<Data>"
  Vector Concatenate/1 -> SPI Controller Transfer/1
  Bus Selector/2 -> MATLAB Function/2(Length)  "<Length>"
  SPI Controller Transfer1/1 -> Terminator1/1
  MATLAB Function/2(CANVector) -> Vector Concatenate/3
  TX Buffer 0/1 -> Vector Concatenate/2
  MATLAB Function/3(RTSByte) -> SPI Controller Transfer1/1
  RTS/1 -> MATLAB Function/4(RTS)
  MCPInitialized/1 -> MATLAB Function/5(MCPInitialized)
  MATLAB Function/1(WriteInstruction) -> Vector Concatenate/1

== system ENV_hardcoded/CAN Tx6 ==
  MCPInitialized : Inport  SampleTime=.001
  BBMSP0A0C : Inport  Port=2
  BBalancingActive : Inport  Port=3
  MTractionControlFLTotal : Inport  Port=4
  MTractionControlFRTotal : Inport  Port=5
  MTractionControlRLTotal : Inport  Port=6
  MTractionControlRRTotal : Inport  Port=7
  NABSMultiplierFL : Inport  Port=8
  NABSMultiplierFR : Inport  Port=9
  Bus Selector : BusSelector  OutputSignals=ID,Length,Data
  CAN Pack : canmsglib/CAN Pack  CANdbFile=C:\Users\William\Downloads\VCUSTM32\BaselineControls\CAN\CAN3_baseline.dbc  MsgList=Etas_Signals_07  MsgName=Etas_Signals_07  MsgIDType=Standard (11-bit identifier)  MsgIdentifier=2035  CANIDInput=off  MsgLength=8  Remote=off  ApplyMinMax=off  BusOutput=on  SignalInfo={'BBMSP0A0C','63','1','LE','unsigned','Standard','0','1','0','0','1';'BBalancingActive','62','1','LE','unsigned','Standard','0','1','0','0','1';'MTractionControlFLTotal','12','12','LE','signed','Standard','0','0.1','50','-Inf','Inf';'MTractionControlFRTotal','24','12','LE','signed','Standard','0','0.1','50','-154.8','254.7';'MTractionControlRLTotal','36','12','LE','signed','Standard','0','0.1','50','-154.8','254.7';'MTractionControlRRTotal','0','12','LE','signed','Standard','0','0.1','50','-154.8','254.7';'NABSMultiplierFL','48','7','LE','unsigned','Standard','0','0.01','0','0','1.27';'NABSMultiplierFR','55','7','LE','unsigned','Standard','0','0.01','0','0','1.27'}
      settings: LibrarySourceBlock=stmutilitieslib/CAN Pack  DataFormat=CANdb specified signals
  MATLAB Function : MATLAB Function  TreatAsAtomicUnit=on
  Offset : Constant  Value=9  OutDataTypeStr=uint16  SampleTime=.001
  Period : Constant  Value=10  OutDataTypeStr=uint16  SampleTime=.001
  RTS : Constant  Value=0x81  OutDataTypeStr=uint8  SampleTime=.001
  SPI Controller Transfer : stm32blockslib/SPI Controller Transfer  Priority=1  SPIModuleSelect=SPI1  ClockPolarity=Low  ClockPhase=1 Edge  SPIModule=uint32(0)  Mode=Master  BusSpeed=uint32(1000000)  FirstBitToTransfer=Most significant bit (MSB)  ClockMode=0  BlockFunction=Transfer  EnableRegisterAddress=off  RegisterAddress=0  OutputDataType=uint8  OutputDataLength=1  OutputStatus=off  BlockingMode=off  Timeout=0.01  DataBits=8  UseCustomSSPin=Explicit GPIO calls  ActiveLowSSPin=Active low  Port_Select=GPIOA  Pin=4
      settings: LibrarySourceBlock=stm32h7xxblockslib/SPI Controller Transfer
  SPI Controller Transfer1 : stm32blockslib/SPI Controller Transfer  Priority=2  SPIModuleSelect=SPI1  ClockPolarity=Low  ClockPhase=1 Edge  SPIModule=uint32(0)  Mode=Master  BusSpeed=uint32(1000000)  FirstBitToTransfer=Most significant bit (MSB)  ClockMode=0  BlockFunction=Transfer  EnableRegisterAddress=off  RegisterAddress=0  OutputDataType=uint8  OutputDataLength=1  OutputStatus=off  BlockingMode=off  Timeout=0.01  DataBits=8  UseCustomSSPin=Explicit GPIO calls  ActiveLowSSPin=Active low  Port_Select=GPIOA  Pin=4
      settings: LibrarySourceBlock=stm32h7xxblockslib/SPI Controller Transfer
  TX Buffer 0 : Constant  Value=0x31  OutDataTypeStr=uint8  SampleTime=.001
  Terminator : Terminator
  Terminator1 : Terminator
  Vector Concatenate : Concatenate  NumInputs=3
  wires:
  BBalancingActive/1 -> CAN Pack/2
  BBMSP0A0C/1 -> CAN Pack/1
  MTractionControlFLTotal/1 -> CAN Pack/3
  MTractionControlFRTotal/1 -> CAN Pack/4
  MTractionControlRLTotal/1 -> CAN Pack/5
  MTractionControlRRTotal/1 -> CAN Pack/6
  NABSMultiplierFL/1 -> CAN Pack/7
  NABSMultiplierFR/1 -> CAN Pack/8
  Bus Selector/2 -> MATLAB Function/2(Length)  "<Length>"
  Vector Concatenate/1 -> SPI Controller Transfer/1
  Bus Selector/1 -> MATLAB Function/1(ID)  "<ID>"
  SPI Controller Transfer/1 -> Terminator/1
  MATLAB Function/1(WriteInstruction) -> Vector Concatenate/1
  MATLAB Function/3(RTSByte) -> SPI Controller Transfer1/1
  RTS/1 -> MATLAB Function/4(RTS)
  SPI Controller Transfer1/1 -> Terminator1/1
  Bus Selector/3 -> MATLAB Function/3(Data)  "<Data>"
  MATLAB Function/2(CANVector) -> Vector Concatenate/3
  CAN Pack/1 -> Bus Selector/1
  TX Buffer 0/1 -> Vector Concatenate/2
  MCPInitialized/1 -> MATLAB Function/5(MCPInitialized)
